simulink model "EnablePort4"  (R2017b)
settings: Solver=FixedStepDiscrete  StartTime=0.0  StopTime=10.0  FixedStep=0.200000  RelTol=1e-3  EnableMultiTasking=on
settings Model: Creator=hbourbou  LastModifiedBy=hbourbou
settings DataIOCC: LimitDataPoints=on
settings OptimizationCC: LifeSpan=inf
settings DebuggingCC: SFUnexpectedBacktrackingDiag=warning  SFNoUnconditionalDefaultTransitionDiag=warning  SFExecutionAtInitializationDiag=none
settings HardwareCC: ProdBitPerSizeT=32  ProdBitPerPtrDiffT=32  ProdWordSize=32  ProdHWDeviceType=Specified
settings ModelReferenceCC: PropagateSignalLabelsOutOfModel=off
settings CodeAppCC: StateflowObjectComments=on
settings GRTTargetCC: TargetLangStandard=C89/C90 (ANSI)
settings ConfigComp: CovMetricSettings=dw  CovHtmlReporting=on  CovSaveCumulativeToWorkspaceVar=on  CovSaveSingleToWorkspaceVar=on  CovExternalEMLEnable=off

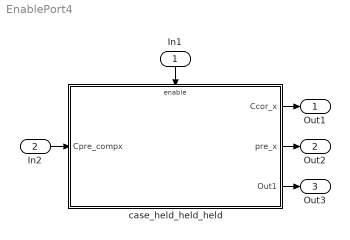
== system EnablePort4 ==
  In1 : Inport
  In2 : Inport  Port=2
  case_held_held_held : Subsystem  TreatAsAtomicUnit=on
  Out1 : Outport
  Out2 : Outport  Port=2
  Out3 : Outport  Port=3
  wires:
  In1/1 -> case_held_held_held/Enable
  case_held_held_held/2(pre_x) -> Out2/1
  case_held_held_held/1(Ccor_x) -> Out1/1
  case_held_held_held/3(Out1) -> Out3/1
  In2/1 -> case_held_held_held/1(Cpre_compx)

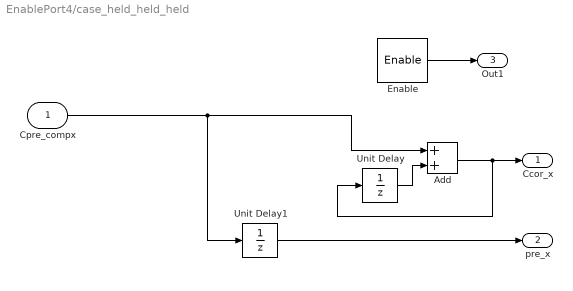
== system EnablePort4/case_held_held_held ==
  Cpre_compx : Inport  OutDataTypeStr=double  PortDimensions=[1]
  Enable : EnablePort  ShowOutputPort=on
  Add : Sum
  Unit Delay : UnitDelay  SampleTime=-1.0000000000000000
  Unit Delay1 : UnitDelay  SampleTime=-1.0000000000000000
  Ccor_x : Outport  InitialOutput=0
  pre_x : Outport  Port=2  InitialOutput=0
  Out1 : Outport  Port=3
  wires:
  Cpre_compx/1 -> Unit Delay1/1, Add/1
  Unit Delay/1 -> Add/2
  Add/1 -> Unit Delay/1, Ccor_x/1
  Enable/1 -> Out1/1
  Unit Delay1/1 -> pre_x/1
